simulink model "Cart_pole_simulation"  (R2025b)
settings: Solver=daessc  StartTime=0.0  StopTime=10  RelTol=1e-3
values from neighbouring files (symbols this model uses):
  N = 40    [cart_pole_ocp.m]    (also in minimal_example_closed_loop.m = 20)
  nu = length(model.u)    [cart_pole_ocp.m]    (also in minimal_example_closed_loop.m = model.u.rows())
  ny_0 = nu    [cart_pole_ocp.m]
  T = 1    [cart_pole_ocp.m]    (also in minimal_example_closed_loop.m = shooting_nodes(end))
undefined symbols (not defined in the file or in its folder): X, Y, Z
libraries: sm_lib x40, nesl_utility x19
(part 2 of 2)

== matlab function Cart_pole_simulation/MATLAB Function ==
  data: ang input; ang_wrapped output
function ang_wrapped = wrapTo2PiCustom(ang)
% wrapTo2PiCustom Envuelve ángulos al rango [0, 2*pi)
%
%   ang_wrapped = wrapTo2PiCustom(ang)
%
%   ang puede ser escalar, vector o matriz (en radianes)

    ang_wrapped = mod(ang, 2*pi);

    % Asegura que 2*pi no aparezca (opcional, por consistencia matemática)
    ang_wrapped(ang_wrapped == 2*pi) = 0;
end
